simulink model "ConfiguredVirtualVehicleModel"  (R2025b)
settings: Solver=ode14x  StartTime=0  StopTime=inf  FixedStep=.001  RelTol=1e-2  EnableMultiTasking=on
StopFcn:
  | %toc
undefined symbols (not defined in the file or in its folder): CtrlTcuInitGear, DriverPreviewDist, EnvAbsPrs, EnvAirTemp, EnvGrvty, EnvNomFrictionScaling, EnvNominalGrade, EnvWindVelX, EnvWindVelY, EnvWindVelZ, MotoFrmInert, MotoFrmLngth, MotoFrmMass, MotoLowrFrntFrkMass, MotoRearArmLngth, MotoRearArmMass, MotoUpprFrntFrkMass, PlntEngTqMax, RiderMass, Sim3dSensor, trackData
libraries: sm_lib x12, simulink x11, nesl_utility x8, sim3dgroundtruthsensorlib x2, autolibshared x2, vehdynlibdriver x2, instrumentseriallib x2, sharedtransform x1, vehdynlibviscommon x1, autolibutils x1, vehdynlibscenariocommon x1, vehdynlibsteering x1
(part 2 of 5)

== system ConfiguredVirtualVehicleModel/Server Communication/Performance Calculations ==
  VehSpd : Inport
  FuelVolFlow : Inport  Port=2
  Integrator : Integrator
  Integrator1 : Integrator
  L/100 Km Calc : Product  Inputs=/*
  Product : Product
  Rate Transition3 : RateTransition  Deterministic=off
  Saturation : Saturate  UpperLimit=Inf  LowerLimit=0.001  ZeroCross=off
  Saturation1 : Saturate  UpperLimit=Inf  LowerLimit=1e-3  ZeroCross=off
  Signal Specification5 : SignalSpecification  Unit=m/s
  Sqrt : Sqrt
  US MPG Calc : Product  Inputs=*/
  Unit Conversion5 : UnitConversion
  m to 100Km : Gain  Gain=1/1000/100
  m to mile : Gain  Gain=0.000621371
  m^3 to L : Gain  Gain=1000
  m^3 to US Gal : Gain  Gain=264.172
  US MPG : Outport  VectorParamsAs1DForOutWhenUnconnected=off
  L/100Km : Outport  Port=2  VectorParamsAs1DForOutWhenUnconnected=off
  wires:
  m^3 to US Gal/1 -> Saturation1/1
  m^3 to L/1 -> L/100 Km Calc/2
  Integrator/1 -> m to mile/1, m to 100Km/1
  m to mile/1 -> US MPG Calc/1
  Integrator1/1 -> m^3 to US Gal/1, m^3 to L/1
  Saturation/1 -> L/100 Km Calc/1
  m to 100Km/1 -> Saturation/1
  L/100 Km Calc/1 -> L/100Km/1  "L/100Km"
  US MPG Calc/1 -> Rate Transition3/1
  Saturation1/1 -> US MPG Calc/2
  Rate Transition3/1 -> US MPG/1  "US MPG"
  FuelVolFlow/1 -> Integrator1/1
  Sqrt/1 -> Integrator/1
  Product/1 -> Sqrt/1
  Signal Specification5/1 -> Product/2, Product/1
  Unit Conversion5/1 -> Signal Specification5/1
  VehSpd/1 -> Unit Conversion5/1

== system ConfiguredVirtualVehicleModel/Visualization/DataLogging ==
  VehFdbk : Inport
  Bus Selector : BusSelector  OutputSignals=Body.Genrl.Vel.xdot,Body.Genrl.Ang.thetafrm,Body.Genrl.AngVel.thetafrmdot,RearArm.Genrl.Ang.thetara,Body.BdyFrm.Cg.Acc.ax,Body.BdyFrm.Cg.Acc.ay,RearArm.Genrl.AngVel.thetaradot,Driveline.EngSpd,Wheels.RearTire.Omega
  Terminator{,1..8} (9 alike) : Terminator
  wires:
  Bus Selector/7 -> Terminator6/1  "<thetaradot>"
  VehFdbk/1 -> Bus Selector/1
  Bus Selector/6 -> Terminator5/1  "<ay>"
  Bus Selector/5 -> Terminator4/1  "<ax>"
  Bus Selector/1 -> Terminator/1  "<xdot>"
  Bus Selector/4 -> Terminator3/1  "<thetara>"
  Bus Selector/3 -> Terminator2/1  "<thetafrmdot>"
  Bus Selector/2 -> Terminator1/1  "<thetafrm>"
  Bus Selector/8 -> Terminator7/1  "<EngSpd>"
  Bus Selector/9 -> Terminator8/1  "<Omega>"

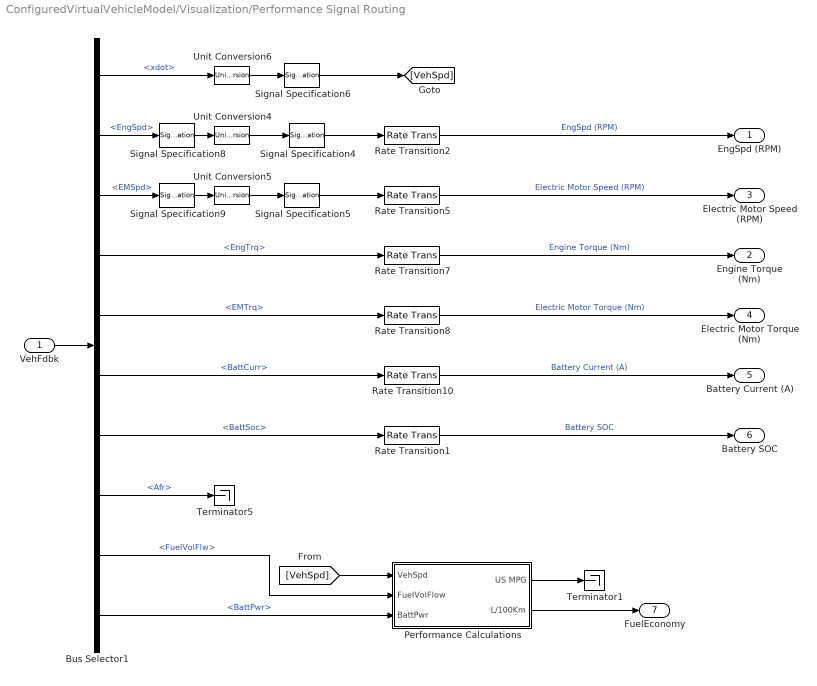
== system ConfiguredVirtualVehicleModel/Visualization/Performance Signal Routing ==
  VehFdbk : Inport
  Bus Selector1 : BusSelector  OutputSignals=Body.BdyFrm.Cg.Vel.xdot,Driveline.EngSpd,Driveline.EMSpd,Engine.EngTrq,ElecMachine.EMTrq,Battery.BattCurr,Battery.BattSoc,Engine.EngineInfo.Afr,Engine.EngineInfo.FuelVolFlw,Battery.BattPwr
  Performance Calculations : Subsystem
  Rate Transition{1..2,5,7..8,10} (6 alike) : RateTransition  Deterministic=off
  Signal Specification4 : SignalSpecification  Unit=rpm
  Signal Specification5 : SignalSpecification  Unit=rpm
  Signal Specification6 : SignalSpecification  Unit=mph
  Signal Specification8 : SignalSpecification  Unit=rad/s
  Signal Specification9 : SignalSpecification  Unit=rad/s
  Terminator1 : Terminator
  Terminator5 : Terminator
  Unit Conversion4 : UnitConversion
  Unit Conversion5 : UnitConversion
  Unit Conversion6 : UnitConversion
  EngSpd (RPM) : Outport
  Engine Torque (Nm) : Outport  Port=2
  Electric Motor Speed (RPM) : Outport  Port=3
  Electric Motor Torque (Nm) : Outport  Port=4
  Battery Current (A) : Outport  Port=5
  Battery SOC : Outport  Port=6
  FuelEconomy : Outport  Port=7
  wires:
  Signal Specification4/1 -> Rate Transition2/1
  Performance Calculations/2(L/100Km) -> FuelEconomy/1
  Bus Selector1/4 -> Rate Transition7/1  "<EngTrq>"
  Bus Selector1/7 -> Rate Transition1/1  "<BattSoc>"
  Signal Specification6/1 -> [VehSpd]
  Bus Selector1/9 -> Performance Calculations/2(FuelVolFlow)  "<FuelVolFlw>"
  Bus Selector1/5 -> Rate Transition8/1  "<EMTrq>"
  Bus Selector1/10 -> Performance Calculations/3(BattPwr)  "<BattPwr>"
  Bus Selector1/2 -> Signal Specification8/1  "<EngSpd>"
  Rate Transition7/1 -> Engine Torque (Nm)/1  "Engine Torque (Nm)"
  Unit Conversion6/1 -> Signal Specification6/1
  Bus Selector1/6 -> Rate Transition10/1  "<BattCurr>"
  Signal Specification5/1 -> Rate Transition5/1
  Unit Conversion5/1 -> Signal Specification5/1
  Unit Conversion4/1 -> Signal Specification4/1
  Signal Specification9/1 -> Unit Conversion5/1
  Signal Specification8/1 -> Unit Conversion4/1
  Bus Selector1/8 -> Terminator5/1  "<Afr>"
  Rate Transition2/1 -> EngSpd (RPM)/1  "EngSpd (RPM)"
  Bus Selector1/3 -> Signal Specification9/1  "<EMSpd>"
  [VehSpd] -> Performance Calculations/1(VehSpd)
  Bus Selector1/1 -> Unit Conversion6/1  "<xdot>"
  Rate Transition8/1 -> Electric Motor Torque (Nm)/1  "Electric Motor Torque (Nm)"
  Rate Transition5/1 -> Electric Motor Speed (RPM)/1  "Electric Motor Speed (RPM)"
  VehFdbk/1 -> Bus Selector1/1
  Rate Transition1/1 -> Battery SOC/1  "Battery SOC"
  Rate Transition10/1 -> Battery Current (A)/1  "Battery Current (A)"
  Performance Calculations/1(US MPG) -> Terminator1/1

== system ConfiguredVirtualVehicleModel/Environment/Friction/Constant Friction ==
  Friction Scaling : Constant  Value=ones(2,1).*EnvNomFrictionScaling  SampleTime=0
  FricCoeffLambda : Outport
  wires:
  Friction Scaling/1 -> FricCoeffLambda/1

== system ConfiguredVirtualVehicleModel/Environment/Friction/Varying Friction ==
  MotoFdbk : Inport
  Bus Selector1 : BusSelector  OutputSignals=Whl.Genrl.Frnt.Cp.Disp.x,Whl.Genrl.Rear.Cp.Disp.x,Whl.Genrl.Frnt.Cp.Disp.y,Whl.Genrl.Rear.Cp.Disp.y
  Bus Selector2 : BusSelector  OutputSignals=Body.InertFrm.Cg.Disp
  Road Track Friction : Subsystem  mask(Road Track Friction){surface_popup=Split friction coefficient scaling factor, lambda_g=EnvNomFrictionScaling, lambda_r=.6, r_x0=175, r_y0=-100, r_xw=1000, r_yw=500, aMode=2}
      mask prompts: surface_popup "vdynblks:vehdynManFriction:blkPrm_surface_popup"; lambda_g "vdynblks:vehdynManFriction:blkPrm_lambda_g"; lambda_r "vdynblks:vehdynManFriction:blkPrm_lambda_r"; r_x0 "vdynblks:vehdynManFriction:blkPrm_r_x0"; r_y0 "vdynblks:vehdynManFriction:blkPrm_r_y0"; r_xw "vdynblks:vehdynManFriction:blkPrm_r_xw"; r_yw "vdynblks:vehdynManFriction:blkPrm_r_yw"
      mask init:
      | % Scaling factor for the friction coefficient around the rectangular region
      | mutable = [lambda_g, lambda_g, lambda_g, lambda_g;
      |            lambda_g, lambda_r, lambda_r, lambda_g; 
      |            lambda_g, lambda_r, lambda_r, lambda_g; 
      |            lambda_g, lambda_g, lambda_g, lambda_g ];
      |        
      | 
      | % The step is distance between breakpoint near the boundary of high and
      | % low friction coefficient
      | 
      | step = 0.01 ; 
      | 
      | % In the mask initialization, xbr and ybr breakpoints are with respect to
      | % Body fixed coordinate system. At time t=0, xbr and ybr breakpoints
      | % updates to Earth (Inertial) Fixed coordinate system. The breakpoints for
      | % the lookup table are added via inputs.
      | 
      | xbr = [(r_x0 - step) , (r_x0 + step), (r_x0 + r_xw - step) , (r_x0 + r_xw + step) ];
      | ybr = [(r_y0 - step) , (r_y0 + step), (r_y0 + r_yw - step) , (r_y0 + r_yw + step) ];
      | 
      | 
      | % To check if the created track is split mu or constant mu
      | 
      | surface_popup = get_param(gcb, 'surface_popup');
      | 
      | if strcmp(surface_popup, 'Split friction coefficient scaling factor')
      |     SplitLambdaTrck = 1;
      | elseif strcmp(surface_popup, 'Constant friction coefficient scaling factor')
      |     SplitLambdaTrck = 0;
      | end
      mask Help: eval('vdynblkshelp(''vdynblkstrack'')');
      mask TypeOptions surface_popup: vdynblks:vehdynManFriction:blkCmb_surface_popup_c1 | vdynblks:vehdynManFriction:blkCmb_surface_popup_c2
      mask Callback surface_popup:
      | surface_popup = get_param(gcb, 'surface_popup');
      | m = Simulink.Mask.get(gcb);
      | 
      | lambda_g = m.getParameter('lambda_g');
      | lambda_r = m.getParameter('lambda_r');
      | r_x0 = m.getParameter('r_x0');
      | r_y0 = m.getParameter('r_y0');
      | r_xw = m.getParameter('r_xw');
      | r_yw = m.getParameter('r_yw');
      | %track_view = m.getParameter('track_view');
      | 
      | 
      | if strcmp(surface_popup, 'Split friction coefficient scaling factor')
      |     lambda_g.Visible = 'on';
      |     lambda_r.Visible = 'on';
      |     r_x0.Visible = 'on';
      |     r_y0.Visible = 'on';
      |     r_xw.Visible = 'on';
      |     r_yw.Visible = 'on';
      |     %track_view.Visible = 'on';
      | 
      | elseif strcmp(surface_popup,'Constant friction coefficient scaling factor')
      |     lambda_g.Visible = 'on';
      |     lambda_r.Visible = 'off';
      |     r_x0.Visible = 'off';
      |     r_y0.Visible = 'off';
      |     r_xw.Visible = 'off';
      |     r_yw.Visible = 'off';
      |     %track_view.Visible = 'off';
      | end
      | [~]=autosharedicon('autolibutils',gcb,0);
      mask DialogControl DescGroupVar Prompt: Road Track Friction
      mask DialogControl DescTextVar Prompt: vdynblks:vehdynManFriction:blkDesc
      mask DialogControl surface_popup Prompt: Type of surface:
      mask DialogControl lambda_g Prompt: Scaling factor for the friction coefficient of ground, lambda_g :
      mask DialogControl lambda_r Prompt: Scaling factor for the friction coefficient of rectangular surface, lambda_r :
      mask DialogControl r_x0 Prompt: X coordinate of lower left corner of rectangular surface, r_x0 [m]:
      mask DialogControl r_y0 Prompt: Y coordinate of lower left corner of rectangular surface, r_y0 [m]:
      mask DialogControl r_xw Prompt: Rectangular surface width in X direction, r_xw [m]:
      mask DialogControl r_yw Prompt: Rectangular surface width in Y direction, r_yw [m]:
  Wheel Coordinates : Subsystem
  FricCoeffLambda : Outport
  wires:
  Wheel Coordinates/1(XWhl) -> Road Track Friction/1(XWhl)
  MotoFdbk/1 -> Bus Selector2/1, Bus Selector1/1
  Wheel Coordinates/2(YWhl) -> Road Track Friction/2(YWhl)
  Road Track Friction/1(FricCoeffLambda) -> FricCoeffLambda/1
  Bus Selector2/1 -> Road Track Friction/3(Cg)  "<Disp>"
  Bus Selector1/1 -> Wheel Coordinates/1(FrntAxlX)  "<x>"
  Bus Selector1/2 -> Wheel Coordinates/2(RearAxlX)  "<x>"
  Bus Selector1/3 -> Wheel Coordinates/3(FrntAxlY)  "<y>"
  Bus Selector1/4 -> Wheel Coordinates/4(RearAxlY)  "<y>"

== system ConfiguredVirtualVehicleModel/Environment/Ground Feedback/3D Engine ==
  Friction : Inport
  WheelFdbk : Inport  Port=2
  3D Engine Source : Subsystem  Variant=on  VariantControl=Choice  mask(Terrain Source){terrType=Single point}
      mask prompts: terrType "Terrain feedback type:"
      mask help:
      | This variant subsystem provides the option for:
      | - a single point of contact for each wheel with minimal post-processing ideal for smooth surfaces and maximum run-time performance.
      | - multiple points of contact per wheel which may be used when interested in non-smooth terrain at a higher computational cost and requires Vehicle Dynamics Blockset.
      mask TypeOptions terrType: Single point | Multiple points
  Bus Creator2 : BusCreator  Inputs=2
  Bus Creator3 : BusCreator  Inputs=3
  Demux1 : Demux  Outputs=2
  Signal Specification1 : SignalSpecification  Unit=1
  Ground : Outport  VectorParamsAs1DForOutWhenUnconnected=off
  wires:
  3D Engine Source/2(DCM) -> Bus Creator3/2  "DCM"
  3D Engine Source/1(z) -> Bus Creator3/1  "z"
  WheelFdbk/1 -> 3D Engine Source/1(WheelFdbk)
  Friction/1 -> Signal Specification1/1
  Bus Creator3/1 -> Ground/1
  Bus Creator2/1 -> Bus Creator3/3  "mu"
  Demux1/2 -> Bus Creator2/2  "mu_R"
  Demux1/1 -> Bus Creator2/1  "mu_F"
  Signal Specification1/1 -> Demux1/1

== system ConfiguredVirtualVehicleModel/Environment/Ground Feedback/Constant ==
  Friction : Inport
  Bus Creator : BusCreator  Inputs=2
  Bus Creator2 : BusCreator  Inputs=2
  Bus Creator3 : BusCreator  Inputs=3
  Constant1 : Constant  Value=zeros(2,1)
  Constant2 : Constant  Value=repmat(eye(3),1,1,2)  SampleTime=-1
  Demux : Demux  Outputs=2
  Demux1 : Demux  Outputs=2
  Signal Specification : SignalSpecification  Unit=m
  Signal Specification1 : SignalSpecification  Unit=1
  Ground : Outport  VectorParamsAs1DForOutWhenUnconnected=off
  wires:
  Constant1/1 -> Signal Specification/1
  Signal Specification/1 -> Demux/1
  Demux/1 -> Bus Creator/1  "G_F_z"
  Demux/2 -> Bus Creator/2  "G_R_z"
  Bus Creator/1 -> Bus Creator3/1  "z"
  Demux1/1 -> Bus Creator2/1  "mu_F"
  Demux1/2 -> Bus Creator2/2  "mu_R"
  Bus Creator2/1 -> Bus Creator3/3  "mu"
  Friction/1 -> Signal Specification1/1
  Signal Specification1/1 -> Demux1/1
  Bus Creator3/1 -> Ground/1
  Constant2/1 -> Bus Creator3/2  "DCM"

== system ConfiguredVirtualVehicleModel/Motorcycle Vehicle/Body, Steer, Suspension, Wheels/Body, Steer, Suspension, Wheels ==
  WindXYZ : Inport
  BrkPrs : Inport  Port=2
  MDrvSprtR : Inport  Port=3
  MDrvArmR : Inport  Port=4
  MDrvFrm : Inport  Port=5
  ScaleFactrs : Inport  Port=6
  SteerCmd : Inport  Port=7
  In_Plane_ModelArchitecture : Subsystem  VariantControl=In_Plane_ModelArchitecture  ReferencedSubsystem=In_Plane_ModelArchitecture
  Moto : Outport
  Wheels : Outport  Port=2

== system ConfiguredVirtualVehicleModel/Motorcycle Vehicle/Body, Steer, Suspension, Wheels/Chassis Input ==
  Env : Inport
  Driveline : Inport  Port=2
  Rider : Inport  Port=3
  Bus Selector : BusSelector  OutputSignals=SteerFdbk
  Bus Selector2 : BusSelector  OutputSignals=Wind,Gnd.mu
  Bus Selector4 : BusSelector  OutputSignals=BrkPrs,Info.ChainInfo.MDrvSprtR,Info.MDrvArmR,Info.MDrvFrm
  Bus to Vector : BusToVector
  Wind : Outport  VectorParamsAs1DForOutWhenUnconnected=off
  BrkPrs : Outport  Port=2  VectorParamsAs1DForOutWhenUnconnected=off
  MDrvSprtR : Outport  Port=3  VectorParamsAs1DForOutWhenUnconnected=off
  MDrvArmR : Outport  Port=4  VectorParamsAs1DForOutWhenUnconnected=off
  MDrvFrm : Outport  Port=5  VectorParamsAs1DForOutWhenUnconnected=off
  ScaleFactrs : Outport  Port=6  VectorParamsAs1DForOutWhenUnconnected=off
  SteerCmd : Outport  Port=7  VectorParamsAs1DForOutWhenUnconnected=off
  wires:
  Env/1 -> Bus Selector2/1
  Bus Selector2/1 -> Wind/1  "<Wind>"
  Driveline/1 -> Bus Selector4/1
  Bus Selector4/4 -> MDrvFrm/1  "<MDrvFrm>"
  Bus Selector4/3 -> MDrvArmR/1  "<MDrvArmR>"
  Bus Selector4/2 -> MDrvSprtR/1  "<MDrvSprtR>"
  Bus Selector4/1 -> BrkPrs/1  "<BrkPrs>"
  Bus Selector2/2 -> Bus to Vector/1  "<mu>"
  Bus to Vector/1 -> ScaleFactrs/1
  Rider/1 -> Bus Selector/1
  Bus Selector/1 -> SteerCmd/1  "<SteerFdbk>"

== system ConfiguredVirtualVehicleModel/Motorcycle Vehicle/Body, Steer, Suspension, Wheels/Chassis Output ==
  Moto : Inport
  Wheels : Inport  Port=2
  Out Bus Element4 : Outport  PortName=MotoFdbk
  Out Bus Element1 : Outport  Port=2  PortName=WheelsFdbk
  wires:
  Moto/1 -> Out Bus Element4/1
  Wheels/1 -> Out Bus Element1/1

== system ConfiguredVirtualVehicleModel/Motorcycle Vehicle/Control Feedback/Variant Subsystem ==
  note: 1) Add Subsystem or Model blocks as valid variant choices.
      | 2) You cannot connect blocks at this level. At simulation, connectivity is automatically
      | determined, based on the active variant and port name matching.
  MotoFdbk : Inport
  IMU_Sensor : Subsystem  VariantControl=IMU_Sensor  ReferencedSubsystem=IMU_Sensor
  No_IMU_Sensor : Subsystem  VariantControl=No_IMU_Sensor  ReferencedSubsystem=No_IMU_Sensor
  IMU : Outport

== system ConfiguredVirtualVehicleModel/Motorcycle Vehicle/Hand Levers and Pedals/Hand Levers and Pedals ==
  note: Placeholder for introducing faults, detailed actuator behavior,
      | interactions of other systems with a human interface such
      | as changes in power steering and braking assistance.
  SteerCmd : Inport
  AccCmd : Inport  Port=2
  DecelCmd : Inport  Port=3
  GearCmd : Inport  Port=4
  BrkPrs : Inport  Port=5
  StrWhlTrq : Inport  Port=6
  Brake Pedal : Subsystem
  Dead Zone3 : DeadZone  LowerValue=-.01  UpperValue=.01  ZeroCross=off
  Terminator : Terminator
  Terminator1 : Terminator
  Twist2Acc : Lookup_n-D  NumberOfTableDimensions=1  BreakpointsForDimension1=[0 1]  Table=[0 1]  ExtrapMethod=Clip  InternalRulePriority=Speed  RndMeth=Simplest
  SteerFdbk : Outport
  AccFdbk : Outport  Port=2
  DecelFdbk : Outport  Port=3
  GearFdbk : Outport  Port=4
  wires:
  SteerCmd/1 -> Dead Zone3/1
  DecelCmd/1 -> Brake Pedal/1(DecelCmd)
  GearCmd/1 -> GearFdbk/1
  BrkPrs/1 -> Terminator/1
  StrWhlTrq/1 -> Terminator1/1
  Brake Pedal/1(DecelFdbk) -> DecelFdbk/1
  Dead Zone3/1 -> SteerFdbk/1
  AccCmd/1 -> Twist2Acc/1
  Twist2Acc/1 -> AccFdbk/1

== system ConfiguredVirtualVehicleModel/Motorcycle Vehicle/Hand Levers and Pedals/Pedal Cluster Input ==
  Rider : Inport
  Driveline : Inport  Port=2
  Bus Selector : BusSelector  OutputSignals=SteerCmd,AccelCmd,DecelCmd,GearCmd
  Bus Selector1 : BusSelector  OutputSignals=EMSpd
  Constant : Constant  Value=0
  SteerCmd : Outport  VectorParamsAs1DForOutWhenUnconnected=off
  AccelCmd : Outport  Port=2  VectorParamsAs1DForOutWhenUnconnected=off
  DecelCmd : Outport  Port=3  VectorParamsAs1DForOutWhenUnconnected=off
  GearCmd : Outport  Port=4  VectorParamsAs1DForOutWhenUnconnected=off
  BrkPrs : Outport  Port=5  VectorParamsAs1DForOutWhenUnconnected=off
  StrWhlTrq : Outport  Port=6  VectorParamsAs1DForOutWhenUnconnected=off
  wires:
  Bus Selector/2 -> AccelCmd/1  "<AccelCmd>"
  Rider/1 -> Bus Selector/1
  Bus Selector/3 -> DecelCmd/1  "<DecelCmd>"
  Bus Selector/4 -> GearCmd/1  "<GearCmd>"
  Bus Selector/1 -> SteerCmd/1  "<SteerCmd>"
  Driveline/1 -> Bus Selector1/1
  Bus Selector1/1 -> BrkPrs/1  "<EMSpd>"
  Constant/1 -> StrWhlTrq/1

== system ConfiguredVirtualVehicleModel/Motorcycle Vehicle/Hand Levers and Pedals/Pedal Cluster Output ==
  SteerFdbk : Inport
  AccFdbk : Inport  Port=2
  DecelFdbk : Inport  Port=3
  GearFdbk : Inport  Port=4
  Bus Creator1 : BusCreator  Inputs=4
  Signal Specification : SignalSpecification  Unit=N*m
  Signal Specification1 : SignalSpecification  Unit=1
  Signal Specification2 : SignalSpecification  Unit=1
  Signal Specification3 : SignalSpecification  Unit=1
  OperatorFdbk : Outport
  wires:
  Signal Specification1/1 -> Bus Creator1/2  "AccFdbk"
  Signal Specification3/1 -> Bus Creator1/4  "GearFdbk"
  AccFdbk/1 -> Signal Specification1/1
  DecelFdbk/1 -> Signal Specification2/1
  GearFdbk/1 -> Signal Specification3/1
  Signal Specification/1 -> Bus Creator1/1  "SteerFdbk"
  SteerFdbk/1 -> Signal Specification/1
  Bus Creator1/1 -> OperatorFdbk/1
  Signal Specification2/1 -> Bus Creator1/3  "DecelFdbk"

== system ConfiguredVirtualVehicleModel/Motorcycle Vehicle/Propulsion System/Actuators ==
  note: 1) Add Subsystem or Model blocks as valid variant choices.
      | 2) You cannot connect blocks at this level. At simulation, connectivity is automatically
      | determined, based on the active variant and port name matching.
  TrqCmd : Inport
  EngSpd : Inport  Port=2
  EMTrqCmd : Inport  Port=3
  EMSpd : Inport  Port=4
  AmbTemp : Inport  Port=5
  MotoMappedEngine : Subsystem  VariantControl=MotoMappedEngine  ReferencedSubsystem=MotoMappedEngine
  Eng : Outport
  Battery : Outport  Port=2
  ElecMachine : Outport  Port=3

== system ConfiguredVirtualVehicleModel/Motorcycle Vehicle/Propulsion System/Electrical System Input ==
  Cntrl : Inport
  Driveline : Inport  Port=2
  Env : Inport  Port=3
  Bus Selector : BusSelector  OutputSignals=VCU.EMTrqCmd
  Bus Selector1 : BusSelector  OutputSignals=EMSpd
  Bus Selector2 : BusSelector  OutputSignals=Temp
  First Order Hold : FirstOrderHold  ErrorTolerance=inf
  EMTrqCmd : Outport  VectorParamsAs1DForOutWhenUnconnected=off
  EMSpd : Outport  Port=2  VectorParamsAs1DForOutWhenUnconnected=off
  AmbTemp : Outport  Port=3  VectorParamsAs1DForOutWhenUnconnected=off
  wires:
  Cntrl/1 -> Bus Selector/1
  Bus Selector/1 -> First Order Hold/1  "<EMTrqCmd>"
  Bus Selector1/1 -> EMSpd/1  "<EMSpd>"
  Env/1 -> Bus Selector2/1
  Bus Selector2/1 -> AmbTemp/1  "<Temp>"
  Driveline/1 -> Bus Selector1/1
  First Order Hold/1 -> EMTrqCmd/1

== system ConfiguredVirtualVehicleModel/Motorcycle Vehicle/Propulsion System/Engine Input ==
  Cntrl : Inport
  Driveline : Inport  Port=2
  Bus Selector : BusSelector  OutputSignals=ECU.EngTrqCmd
  Bus Selector1 : BusSelector  OutputSignals=EngSpd
  First Order Hold : FirstOrderHold  OutputAlgorithm=Fast (Minimize Error)  ErrorTolerance=.001
  Rate Transition : RateTransition  OutPortSampleTime=0.001
  EngTrqCmd : Outport  VectorParamsAs1DForOutWhenUnconnected=off
  EngSpd : Outport  Port=2  VectorParamsAs1DForOutWhenUnconnected=off
  wires:
  Driveline/1 -> Bus Selector1/1
  Cntrl/1 -> Bus Selector/1
  Bus Selector/1 -> Rate Transition/1  "<EngTrqCmd>"
  Bus Selector1/1 -> EngSpd/1  "<EngSpd>"
  First Order Hold/1 -> EngTrqCmd/1
  Rate Transition/1 -> First Order Hold/1

== system ConfiguredVirtualVehicleModel/Motorcycle Vehicle/Transmission, Driveline and Brakes/Brake Hydraulics ==
  BrkPrsCmd : Inport
  Front Bias : Constant
  Gain4 : Gain  Gain=8e6
  Mux : Mux  Inputs=2
  Product : Product
  Rear Bias : Constant  Value=.6
  Valve : autolibutils/Cont LPF  wc=20*2*pi  AbsoluteTolerance=auto  aMode=2
  BrkPrs : Outport  VectorParamsAs1DForOutWhenUnconnected=off
  wires:
  Valve/1 -> Product/2
  Gain4/1 -> BrkPrs/1
  BrkPrsCmd/1 -> Valve/1
  Front Bias/1 -> Mux/1
  Rear Bias/1 -> Mux/2
  Product/1 -> Gain4/1
  Mux/1 -> Product/1

== system ConfiguredVirtualVehicleModel/Motorcycle Vehicle/Transmission, Driveline and Brakes/Driveline Input ==
  Cntrl : Inport
  EngTrqCmd : Inport  Port=2
  Wheels : Inport  Port=3
  Moto : Inport  Port=4
  EMTrqCmd : Inport  Port=5
  Bus Selector : BusSelector  OutputSignals=EngTrq
  Bus Selector1 : BusSelector  OutputSignals=EMTrq
  Bus Selector2 : BusSelector  OutputSignals=RearTire.Fx,RearTire.MBrk,RearTire.Omegadot
  Bus Selector3 : BusSelector  OutputSignals=Transmission.GearCmd,VCU.VcuBrkPrsCmd
  Bus Selector5 : BusSelector  OutputSignals=Frame.Genrl.Ang.thetafrm,RearArm.Genrl.Ang.thetara
  Data Type Conversion : DataTypeConversion  SaturateOnIntegerOverflow=off  RndMeth=Floor
  First Order Hold1 : FirstOrderHold  OutputAlgorithm=Fast (Minimize Error)  ErrorTolerance=.001
  First Order Hold2 : FirstOrderHold  InitialOutput=CtrlTcuInitGear  ErrorTolerance=.5
  EngTrq : Outport  VectorParamsAs1DForOutWhenUnconnected=off
  GearCmd : Outport  Port=2  VectorParamsAs1DForOutWhenUnconnected=off
  FCpR. : Outport  Port=3  VectorParamsAs1DForOutWhenUnconnected=off
  ThetaFrm. : Outport  Port=4  VectorParamsAs1DForOutWhenUnconnected=off
  ThetaArmR. : Outport  Port=5  VectorParamsAs1DForOutWhenUnconnected=off
  MBrkR. : Outport  Port=6  VectorParamsAs1DForOutWhenUnconnected=off
  AngAWhlR. : Outport  Port=7  VectorParamsAs1DForOutWhenUnconnected=off
  EMTrq : Outport  Port=8  VectorParamsAs1DForOutWhenUnconnected=off
  BrkPrsCmd : Outport  Port=9  VectorParamsAs1DForOutWhenUnconnected=off
  wires:
  Wheels/1 -> Bus Selector2/1
  Moto/1 -> Bus Selector5/1
  Bus Selector2/3 -> AngAWhlR./1  "<Omegadot>"
  Bus Selector2/2 -> MBrkR./1  "<MBrk>"
  Bus Selector2/1 -> FCpR./1  "<Fx>"
  Bus Selector5/2 -> ThetaArmR./1  "<thetara>"
  Bus Selector5/1 -> ThetaFrm./1  "<thetafrm>"
  EngTrqCmd/1 -> Bus Selector/1
  EMTrqCmd/1 -> Bus Selector1/1
  Bus Selector3/2 -> First Order Hold1/1  "<VcuBrkPrsCmd>"
  Bus Selector3/1 -> Data Type Conversion/1  "<GearCmd>"
  Cntrl/1 -> Bus Selector3/1
  Bus Selector/1 -> EngTrq/1  "<EngTrq>"
  Bus Selector1/1 -> EMTrq/1  "<EMTrq>"
  First Order Hold1/1 -> BrkPrsCmd/1
  Data Type Conversion/1 -> First Order Hold2/1
  First Order Hold2/1 -> GearCmd/1

== system ConfiguredVirtualVehicleModel/Motorcycle Vehicle/Transmission, Driveline and Brakes/Driveline Output ==
  EngSpd : Inport
  Gear : Inport  Port=2
  Info : Inport  Port=3
  EMSpd : Inport  Port=4
  BrkPrs : Inport  Port=5
  Bus Creator1 : BusCreator  Inputs=7
  Ground{,1..3} (4 alike) : Ground
  Mux : Mux  Inputs=2
  Mux1 : Mux  Inputs=2
  Signal Specification7 : SignalSpecification  Unit=Pa  Dimensions=2
  Driveline : Outport  VectorParamsAs1DForOutWhenUnconnected=off
  wires:
  Bus Creator1/1 -> Driveline/1  "Driveline"
  EngSpd/1 -> Bus Creator1/3  "EngSpd"
  EMSpd/1 -> Bus Creator1/2  "EMSpd"
  Gear/1 -> Bus Creator1/4  "Gear"
  Info/1 -> Bus Creator1/7  "Info"
  Mux/1 -> Bus Creator1/6  "AxlTrq"
  Mux1/1 -> Bus Creator1/5  "PropShftSpd"
  Ground3/1 -> Mux/2
  Ground2/1 -> Mux/1
  Ground/1 -> Mux1/1
  Ground1/1 -> Mux1/2
  BrkPrs/1 -> Signal Specification7/1
  Signal Specification7/1 -> Bus Creator1/1  "BrkPrs"

== system ConfiguredVirtualVehicleModel/Motorcycle Vehicle/Transmission, Driveline and Brakes/Transmission and Driveline ==
  EngTrq : Inport
  GearCmd : Inport  Port=2
  FCpR : Inport  Port=3
  ThetaFrm : Inport  Port=4
  ThetaArmR : Inport  Port=5
  MBrkR : Inport  Port=6
  AngAWhlR : Inport  Port=7
  EMTrq : Inport  Port=8
  Driveline : Subsystem  Variant=on  VariantChoicesSpecifier={'Chain_Drive'}  VariantControlMode=label  VariantControl=Choice  LabelModeActiveChoice=Chain_Drive
  Transmission : Subsystem  Variant=on  VariantChoicesSpecifier={'ConventionalMotorcycle'}  VariantControlMode=label  VariantControl=Choice  LabelModeActiveChoice=ConventionalMotorcycle
  EngSpd : Outport
  Gear : Outport  Port=2
  Info : Outport  Port=3
  EMSpd : Outport  Port=4
  wires:
  EngTrq/1 -> Transmission/1(EngTrq)
  GearCmd/1 -> Transmission/2(GearCmd)
  FCpR/1 -> Driveline/1(FCpR)
  ThetaFrm/1 -> Driveline/2(ThetaFrm)
  ThetaArmR/1 -> Driveline/3(ThetaArmR)
  MBrkR/1 -> Driveline/4(MBrkR)
  AngAWhlR/1 -> Driveline/5(AngAWhlR)
  EMTrq/1 -> Transmission/3(EMTrq)
  Driveline/2(DrvSprktSpd) -> Transmission/4(DrvSprktSpd)
  Transmission/4(DrvSprktTrq) -> Driveline/6(DrvSprktTrq)
  Driveline/1(Info) -> Info/1
  Transmission/1(EngSpd) -> EngSpd/1
  Transmission/2(Gear) -> Gear/1
  Transmission/3(EMSpd) -> EMSpd/1

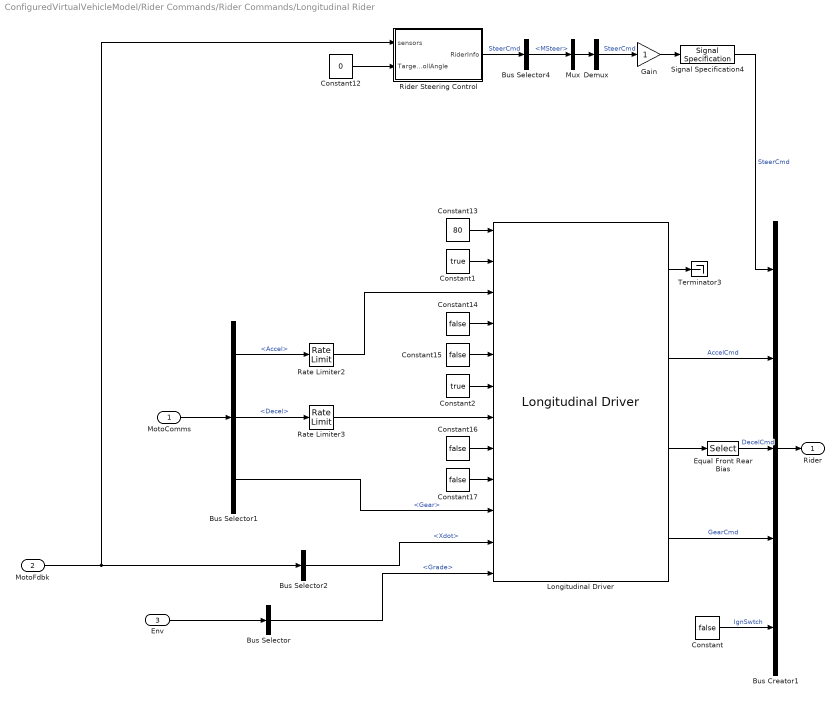
== system ConfiguredVirtualVehicleModel/Rider Commands/Rider Commands/Longitudinal Rider ==
  MotoComms : Inport
  MotoFdbk : Inport  Port=2
  Env : Inport  Port=3
  Bus Creator1 : BusCreator  Inputs=5
  Bus Selector : BusSelector  OutputSignals=Grade
  Bus Selector1 : BusSelector  OutputSignals=Accel,Decel,Gear
  Bus Selector2 : BusSelector  OutputSignals=Body.InertFrm.Cg.Vel.Xdot
  Bus Selector4 : BusSelector  OutputSignals=MSteer
  Constant{,14..17} (5 alike) : Constant  Value=false
  Constant1 : Constant  Value=true
  Constant12 : Constant  Value=0
  Constant13 : Constant  Value=80
  Constant2 : Constant  Value=true
  Demux : Demux  Outputs=1
  Equal Front Rear Bias : Selector  InputPortWidth=1  IndexOptions=Index vector (dialog)  Indices=[1 1]  OutputSizes=1
  Gain : Gain
  Longitudinal Driver : autolibshared/Longitudinal Driver  extAccelOvr=on  extDecelOvr=on  extAccelHld=on  extDecelHld=on  extAccelZero=on  extDecelZero=on  cntrlType=PI  shftType=External  velUnits=m/s  gearOut=on  Kp=5  Ki=5  Kff=.1  Kg=0  VehVelVec=[0 100]  KffVec=[.1 .1]  KpVec=[10 10]  KiVec=[5 5]  KgVec=[0 0]  m=MotoFrmMass+MotoUpprFrntFrkMass+MotoLowrFrntFrkMass+MotoRearArmMass+RiderMass  Kpt=DriverTractiveForce  tau=DriverTimeConst  L=DriverPreviewDist  aR=DriverRollRes  bR=DriverDrivelineRes  cR=DriverAeroRes  g=EnvGrvty  vnom=5  Kaw=1  tauerr=.1  tauPt=2  GearInit=DriverInitialGear  tShift=DriverShiftTime  pdlVec=[0.1 0.4 0.5 0.9]  upShftTbl=|  dwnShftTbl=|  tClutch=.5  tRev=.5  tPark=120  aMode=6  UpGearVec="[0  1  2  3  4  5  6  7  8]"  DownGearVec="[1  2  3  4  5  6  7  8  9]"
      upShftTbl=|
      | [-1 25 42.7198903036173	47.4101666153559	56.5501922484876	82.5161741607935	103.519768418748	161.279652628121	247.919478942182;
      | -1 35 47.2198903036173	51.9101666153559	61.0501922484876	87.0161741607935	108.019768418748	165.779652628121	252.419478942182;
      | -1 40 48.7198903036173	53.4101666153559	62.5501922484876	88.5161741607935	109.519768418748	167.279652628121	253.919478942182;
      | -1 45 54.7198903036173	59.4101666153559	68.5501922484876	94.5161741607935	115.519768418748	173.279652628121	259.919478942182].*0.277778
      dwnShftTbl=|
      | [6 20 38.7198903036173	43.4101666153559	52.5501922484876	78.5161741607935	99.5197684187476	157.279652628121	243.919478942182;
      | 6 30 43.2198903036173	47.9101666153559	57.0501922484876	83.0161741607935	104.019768418748	161.779652628121	248.419478942182;
      | 6 35 44.7198903036173	49.4101666153559	58.5501922484876	84.5161741607935	105.519768418748	163.279652628121	249.919478942182;
      | 6 45 50.7198903036173	55.4101666153559	64.5501922484876	90.5161741607935	111.519768418748	169.279652628121	255.919478942182].*0.277778
  Mux : Mux  Inputs=1
  Rate Limiter2 : RateLimiter  RisingSlewLimit=2  FallingSlewLimit=-5  SampleTimeMode=inherited
  Rate Limiter3 : RateLimiter  RisingSlewLimit=2  FallingSlewLimit=-5  SampleTimeMode=inherited
  Rider Steering Control : Subsystem  mask{RiderControlTypePanel=Roll angle control, TrajectoryTypePanel=Oval, RidTrajContG=0.11, RidTrajContGphi=-21.5, RidTrajContGphid=9, RidTrajContGl=1.7, RidTrajContTD=0.1, RidTrajContTL=0.1, RidRollContGphi=-21.5, RidRollContGphid=9, Trajr=15, Trajl=80, Trajpointdist=1, TrajDatFile='Traj.mat'}
      mask prompts: RiderControlTypePanel "Rider control type:"; TrajectoryTypePanel "Trajectory type:"; RidTrajContG "Gain to determine the Target roll angle, RidContG [rad/m]:"; RidTrajContGphi "Gain to follow the Target trajectory, RidContGphi [Nm/rad]:"; RidTrajContGphid "Gain to prevent the vehicle from tipping over, RidContGphid [Nms/rad]:"; RidTrajContGl "Gain that determines the distance to the look ahead point, RidContGl [s]:"; RidTrajContTD "Time constant for 1st order delay, RidContTD [s]:"; RidTrajContTL "Dead time of rider operation, RidContTL [s]:"; RidRollContGphi "Gain to follow the Target trajectory, RidContGphi [Nm/rad]:"; RidRollContGphid "Gain to prevent the vehicle from tipping over, RidContGphid [Nms/rad]:"; Trajr "Trajectory parameter,Trajr [m]:"; Trajl "Trajectory parameter,Trajl [m]:"; Trajpointdist "Trajpdist [m]:"; TrajDatFile "Trajectory data file:"
      mask init:
      | maskObj = Simulink.Mask.get(gcb);
      | 
      | Type_tmp = maskObj.getParameter('RiderControlTypePanel');
      | Type     = Type_tmp.Value;
      | 
      | TrajGroup = maskObj.getDialogControl('RiderTrajectoryControlParamPanel');
      | RollGroup = maskObj.getDialogControl('RiderRollControlParamPanel');
      | 
      | TrajectoryTypePanel = maskObj.getDialogControl('TrajectoryTypeCont');
      | TargetTrajectoryParamGroup = maskObj.getDialogControl('TargetTrajectoryParamGroup');
      | 
      | GroupAll = maskObj.getDialogControl('RiderControlParamGroup');
      | 
      | switch Type
      |     case 'Roll angle control'
      |     TrajGroup.Visible = 'off';
      |     RollGroup.Visible = 'on';
      |     GroupAll.Visible = 'on';
      |     TrajectoryTypePanel.Visible = 'off';
      |     TargetTrajectoryParamGroup.Visible = 'off';
      |     InputConnector('TargetRollAngle','on');
      |     case 'Target trajectory driving - Look ahead point'
      |     TrajGroup.Visible = 'on';
      |     RollGroup.Visible = 'off';
      |     GroupAll.Visible = 'on';
      |     TrajectoryTypePanel.Visible = 'on';
      |     TargetTrajectoryParamGroup.Visible = 'on';
      |     InputConnector('TargetRollAngle','off','Ground');
      | end
      | 
      | switch Type
      |     case 'Oval'
      | % ------------------------------------------------------------------------%
      | %  Create Trajectory
      | % ------------------------------------------------------------------------%
      | % --- Oval --- %
      | % top part %
      | x_straight1 = -Trajl/2:Trajpointdist:Trajl/2;
      | y_straight1 = x_straight1*0;
      | 
      | % bottom part %
      | x_straight2 = -Trajl/2:Trajpointdist:Trajl/2;
      | y_straight2 = x_straight1*0+2*Trajr;
      | 
      | % right part %
      | theta_corner1 = -pi/2:Trajpointdist/Trajr:pi/2;
      | x_corner1     = Trajr*cos(theta_corner1)+Trajl/2;
      | y_corner1     = Trajr*sin(theta_corner1)+Trajr;
      | 
      | % left part %
      | theta_corner2 = pi/2:Trajpointdist/Trajr:3/2*pi;
      | x_corner2     = Trajr*cos(theta_corner2)-Trajl/2;
      | y_corner2     = Trajr*sin(theta_corner2)+Trajr;
      | 
      | % total %
      | x_oval = [x_straight1, x_corner1(2:end), fliplr(x_straight2), x_corner2(2:end)];
      | y_oval = [y_straight1, y_corner1(2:end), fliplr(y_straight2), y_corner2(2:end)];
      | 
      | trackData(1,:) = x_oval;
      | trackData(2,:) = y_oval;
      | trackData(3,:) = y_oval*0;
      | 
      |     case 'User defined'
      | 
      | TmpTraj = load(TrajDatFile);
      | 
      | trackData(1,:) = TmpTraj.TrajX;
      | trackData(2,:) = -TmpTraj.TrajY;
      | trackData(3,:) = TmpTraj.TrajY*0;
      | 
      | end
      mask Callback RiderControlTypePanel:
      | maskObj = Simulink.Mask.get(gcb);
      | 
      | Type_tmp = maskObj.getParameter('RiderControlTypePanel');
      | Type     = Type_tmp.Value;
      | 
      | TrajGroup = maskObj.getDialogControl('RiderTrajectoryControlParamPanel');
      | RollGroup = maskObj.getDialogControl('RiderRollControlParamPanel');
      | 
      | TrajectoryTypePanel = maskObj.getDialogControl('TrajectoryTypeCont');
      | TargetTrajectoryParamGroup = maskObj.getDialogControl('TargetTrajectoryParamGroup');
      | 
      | GroupAll = maskObj.getDialogControl('RiderControlParamGroup');
      | 
      | switch Type
      |     case 'Roll angle control'
      |     set_param([gcb,'/Rider Steering'],'RiderControlTypePanel','Roll angle control')
      |     TrajGroup.Visible = 'off';
      |     RollGroup.Visible = 'on';
      |     GroupAll.Visible = 'on';
      |     TrajectoryTypePanel.Visible = 'off';
      |     TargetTrajectoryParamGroup.Visible = 'off';
      |     InputConnector('TargetRollAngle','on');
      |     case 'Target trajectory driving - Look ahead point'
      |     set_param([gcb,'/Rider Steering'],'RiderControlTypePanel','Target trajectory driving - Look ahead point')
      |     TrajGroup.Visible = 'on';
      |     RollGroup.Visible = 'off';
      |     GroupAll.Visible = 'on';
      |     TrajectoryTypePanel.Visible = 'on';
      |     TargetTrajectoryParamGroup.Visible = 'on';
      |     InputConnector('TargetRollAngle','off','Ground');
      | end
      mask TypeOptions TrajectoryTypePanel: Oval | User defined
      mask Callback TrajectoryTypePanel:
      | maskObj = Simulink.Mask.get(gcb);
      | 
      | Type_tmp = maskObj.getParameter('TrajectoryTypePanel');
      | Type = Type_tmp.Value;
      | 
      | TargetTrajectoryParamOvalPanel = maskObj.getDialogControl('TargetTrajectoryParamOvalPanel');
      | 
      | TargetTrajectoryParamUserDefinedPanel = maskObj.getDialogControl('TargetTrajectoryParamUserDefinedPanel');
      | 
      | TargetTrajectoryParamGroup = maskObj.getDialogControl('TargetTrajectoryParamGroup');
      | 
      | switch Type
      |     case 'Oval'
      |         set_param([gcb,'/Rider Steering'],'TrajectoryTypePanel','Oval')
      |         % TargetTrajectoryParamGroup.Visible = 'on';
      |         TargetTrajectoryParamOvalPanel.Visible = 'on';
      |         TargetTrajectoryParamUserDefinedPanel.Visible = 'off';
      |     case 'User defined'
      |     set_param([gcb,'/Rider Steering'],'TrajectoryTypePanel','User defined')
      |         % TargetTrajectoryParamGroup.Visible = 'on';
      |         TargetTrajectoryParamOvalPanel.Visible = 'off';
      |         TargetTrajectoryParamUserDefinedPanel.Visible = 'on';
      | end
      mask DialogControl RiderOptionsGroup Prompt: Options
      mask DialogControl RiderTrajectoryControlParamPanel Prompt: Control parameters
      mask DialogControl RiderRollControlParamPanel Prompt: Control parameters
      mask DialogControl TargetTrajectoryParamOvalPanel Prompt: Trajectory parameters
      mask DialogControl OvalTrajConfBtn Prompt: Confirm
      mask DialogControl OvalTrajConfBtn Callback:
      | maskObj = Simulink.Mask.get(gcb);
      | 
      | Trajr_tmp          = maskObj.getParameter('Trajr');
      | Trajr              = str2num(Trajr_tmp.Value);
      | Trajl_tmp          = maskObj.getParameter('Trajl');
      | Trajl              = str2num(Trajl_tmp.Value);
      | Trajpointdist_tmp  = maskObj.getParameter('Trajpointdist');
      | Trajpointdist      = str2num(Trajpointdist_tmp.Value);
      | 
      | % ------------------------------------------------------------------------%
      | %  Create Trajectory
      | % ------------------------------------------------------------------------%
      | % --- Oval --- %
      | % top part %
      | x_straight1 = -Trajl/2:Trajpointdist:Trajl/2;
      | y_straight1 = x_straight1*0;
      | 
      | % bottom part %
      | x_straight2 = -Trajl/2:Trajpointdist:Trajl/2;
      | y_straight2 = x_straight1*0+2*Trajr;
      | 
      | % right part %
      | theta_corner1 = -pi/2:Trajpointdist/Trajr:pi/2;
      | x_corner1     = Trajr*cos(theta_corner1)+Trajl/2;
      | y_corner1     = Trajr*sin(theta_corner1)+Trajr;
      | 
      | % left part %
      | theta_corner2 = pi/2:Trajpointdist/Trajr:3/2*pi;
      | x_corner2     = Trajr*cos(theta_corner2)-Trajl/2;
      | y_corner2     = Trajr*sin(theta_corner2)+Trajr;
      | 
      | % total %
      | x_oval = [x_straight1, x_corner1(2:end), fliplr(x_straight2), x_corner2(2:end)];
      | y_oval = [y_straight1, y_corner1(2:end), fliplr(y_straight2), y_corner2(2:end)];
      | 
      | figure;
      | plot(x_oval, -y_oval);
      | axis equal;
      | grid on;
      | xlabel('Coordinate X [m]');
      | ylabel('Coordinate Y [m]');
      | title('Oval target trajectory');
      | set(gca,'YDir','reverse')
      mask DialogControl TargetTrajectoryParamUserDefinedPanel Prompt: Trajectory parameters
      mask DialogControl UserDefinedTrajConfBtn Prompt: Confirm
      mask DialogControl UserDefinedTrajConfBtn Callback:
      | maskObj = Simulink.Mask.get(gcb);
      | 
      | File_tmp = maskObj.getParameter('TrajDatFile');
      | File     = replace(File_tmp.Value,'''','');
      | 
      | TmpTraj = load(File);
      | 
      | figure;
      | plot(TmpTraj.TrajX, TmpTraj.TrajY);
      | grid on;
      | axis equal;
      | xlabel('Coordinate X [m]');
      | ylabel('Coordinate Y [m]');
      | title('User defined target trajectory');
      | set(gca,'YDir','reverse');
  Signal Specification4 : SignalSpecification  Unit=N*m
  Terminator3 : Terminator
  Rider : Outport  VectorParamsAs1DForOutWhenUnconnected=off
  wires:
  Bus Creator1/1 -> Rider/1
  Longitudinal Driver/3 -> Equal Front Rear Bias/1
  Longitudinal Driver/1 -> Terminator3/1
  MotoComms/1 -> Bus Selector1/1
  Longitudinal Driver/2 -> Bus Creator1/2  "AccelCmd"
  Longitudinal Driver/4 -> Bus Creator1/4  "GearCmd"
  Constant/1 -> Bus Creator1/5  "IgnSwtch"
  Constant2/1 -> Longitudinal Driver/6
  Env/1 -> Bus Selector/1
  Equal Front Rear Bias/1 -> Bus Creator1/3  "DecelCmd"
  Constant1/1 -> Longitudinal Driver/2
  Bus Selector/1 -> Longitudinal Driver/12  "<Grade>"
  Rider Steering Control/1(RiderInfo) -> Bus Selector4/1  "SteerCmd"
  Bus Selector4/1 -> Mux/1  "<MSteer>"
  Signal Specification4/1 -> Bus Creator1/1  "SteerCmd"
  Gain/1 -> Signal Specification4/1
  Demux/1 -> Gain/1  "SteerCmd"
  MotoFdbk/1 -> Rider Steering Control/1(sensors), Bus Selector2/1
  Constant12/1 -> Rider Steering Control/2(TargetRollAngle)
  Mux/1 -> Demux/1
  Constant13/1 -> Longitudinal Driver/1
  Bus Selector2/1 -> Longitudinal Driver/11  "<Xdot>"
  Bus Selector1/3 -> Longitudinal Driver/10  "<Gear>"
  Bus Selector1/1 -> Rate Limiter2/1  "<Accel>"
  Bus Selector1/2 -> Rate Limiter3/1  "<Decel>"
  Constant14/1 -> Longitudinal Driver/4
  Constant15/1 -> Longitudinal Driver/5
  Constant16/1 -> Longitudinal Driver/8
  Constant17/1 -> Longitudinal Driver/9
  Rate Limiter2/1 -> Longitudinal Driver/3
  Rate Limiter3/1 -> Longitudinal Driver/7

== system ConfiguredVirtualVehicleModel/Rider Commands/Rider Commands/Open Loop ==
  MotoFdbk : Inport
  MotoComms : Inport  Port=2
  GearCmd : Inport  Port=3
  Bus Creator1 : BusCreator  Inputs=5
  Bus Selector1 : BusSelector  OutputSignals=SteerOvrCmd,AccelOvrCmd,DecelOvrCmd
  Constant : Constant  Value=false
  Equal Front Rear Bias : Selector  InputPortWidth=1  IndexOptions=Index vector (dialog)  Indices=[1 1]  OutputSizes=1
  Gain : Gain
  Signal Specification : SignalSpecification  Unit=1
  Signal Specification1 : SignalSpecification  Unit=1
  Signal Specification2 : SignalSpecification  Unit=1
  Signal Specification3 : SignalSpecification  Unit=rad
  Signal Specification4 : SignalSpecification  Unit=N*m
  Terminator : Terminator
  Rider : Outport  VectorParamsAs1DForOutWhenUnconnected=off
  wires:
  Signal Specification2/1 -> Bus Creator1/4  "GearCmd"
  Bus Selector1/3 -> Signal Specification1/1  "<DecelOvrCmd>"
  Bus Creator1/1 -> Rider/1
  Bus Selector1/2 -> Signal Specification/1  "<AccelOvrCmd>"
  MotoFdbk/1 -> Terminator/1
  Signal Specification/1 -> Bus Creator1/2  "AccelCmd"
  Equal Front Rear Bias/1 -> Bus Creator1/3  "DecelCmd"
  Constant/1 -> Bus Creator1/5  "IgnSwtch"
  MotoComms/1 -> Bus Selector1/1
  GearCmd/1 -> Signal Specification2/1
  Bus Selector1/1 -> Signal Specification3/1  "<SteerOvrCmd>"
  Signal Specification4/1 -> Bus Creator1/1  "SteerCmd"
  Signal Specification1/1 -> Equal Front Rear Bias/1  "DecelCmd"
  Signal Specification3/1 -> Gain/1
  Gain/1 -> Signal Specification4/1

== system ConfiguredVirtualVehicleModel/Rider Commands/Rider Commands/Predictive Rider ==
  MotoComms : Inport
  MotoFdbk : Inport  Port=2
  Env : Inport  Port=3
  Bus Creator1 : BusCreator  Inputs=5
  Bus Selector : BusSelector  OutputSignals=Body.InertFrm.Cg.Disp.Y,Body.BdyFrm.Cg.Vel.ydot,Body.InertFrm.Cg.Ang.psi,Body.BdyFrm.Cg.AngVel.r
  Bus Selector1 : BusSelector  OutputSignals=LngRef,LtrlRef,EnblSteerCmd,SteerOvrCmd,SteerHld,SteerZero,EnblAccelOvr,AccelOvrCmd,AccelHld,AccelZero,EnblDecelCmd,DecelOvrCmd,DecelHld,DecelZero
  Constant : Constant  Value=false
  Equal Front Rear Bias : Selector  InputPortWidth=1  IndexOptions=Index vector (dialog)  Indices=[1 1]  OutputSizes=1
  Gain : Gain
  Hill Hold : Subsystem
  Linear Predictive Driver : vehdynlibdriver/Predictive Driver  extAccelOvr=on  extDecelOvr=on  extAccelHld=on  extDecelHld=on  extAccelZero=on  extDecelZero=on  extSteerOvr=on  extSteerHld=on  extSteerZero=on  cntrlType=Predictive  cntrlTypeLat=Predictive  shftType=Reverse, Neutral, Drive  coordMode=SAE J670 (Z-down)  refType=Reference pose  velUnits=m/s  angUnits=rad  gearOut=on  steerOut=on  Kp=3  Ki=1  Kff=1  Kg=0  VehVelVec=[0 100]  KffVec=[.1 .1]  KpVec=[10 10]  KiVec=[5 5]  KgVec=[0 0]  vnom=5  Kaw=1  tauerr=.075  tau=DriverTimeConst  L=DriverPreviewDist  Kpt=DriverTractiveForce  aR=DriverRollRes  bR=DriverDrivelineRes  cR=DriverAeroRes  g=EnvGrvty  vecPose=off  dynamMode=off  PositionGainF=2.5  PositionGainR=2.5  YawRateGain=.2  DelayGain=.2  enableDrift=off  BetaRef=10  KpBeta=1  KpDrift=1  KdDrift=1  KpPsi=1  KOmega=.1  tOmega=.1  a=MotoFrmLngth  b=MotoRearArmLngth  m=MotoFrmMass+MotoUpprFrntFrkMass+MotoLowrFrntFrkMass+MotoRearArmMass+RiderMass  Cy_f=DriverFrontCornerStiff  Cy_r=DriverRearCornerStiff  I=MotoFrmInert(3)  Ksteer=1  theta=DriverWheelRange  Idl=1  Re=PlntWhlLdRadius  lambda_mu=1  GearInit=DriverInitialGear  tShift=DriverShiftTime  pdlVec=[0.1 0.4 0.5 0.9]  upShftTbl=[-1 12.9375 26.4375 39.9375 51.18749999999999 62.4375 72.84375 83.25;-1 16.3125 29.8125 43.3125 54.5624 65.8125 76.78125 87.75;-1 19.6875 33.1875 46.68749999999999 57.9375 69.1875 80.71875 92.25;-1 33 52.5 77.25 100.5 138.75 161.875 185]  dwnShftTbl=[-1 12.9375 26.4375 39.9375 51.18749999999999 62.4375 72.84375 83.25;-1 16.3125 29.8125 43.3125 54.5624 65.8125 76.78125 87.75;-1 19.6875 33.1875 46.68749999999999 57.9375 69.1875 80.71875 92.25;-1 33 52.5 77.25 100.5 138.75 161.875 185]  tClutch=.5  tRev=.5  tPark=120  UpGearVec="[0  1  2  3  4  5  6  7]"  DownGearVec="[1  2  3  4  5  6  7  8]"  aMode=2
  Signal Specification4 : SignalSpecification  Unit=N*m
  Terminator : Terminator
  Unit Conversion : UnitConversion
  " Rider" : Outport  VectorParamsAs1DForOutWhenUnconnected=off
  wires:
  Linear Predictive Driver/3 -> Bus Creator1/2  "AccelCmd"
  Bus Selector/2 -> Linear Predictive Driver/18  "<ydot>"
  Bus Selector/1 -> Linear Predictive Driver/17  "<Y>"
  Bus Selector1/10 -> Linear Predictive Driver/10  "<AccelZero>"
  Bus Creator1/1 -> " Rider"/1
  Linear Predictive Driver/1 -> Terminator/1
  Bus Selector/3 -> Linear Predictive Driver/19  "<psi>"
  MotoFdbk/1 -> Hill Hold/7(VehFdbk), Bus Selector/1
  Bus Selector1/2 -> Linear Predictive Driver/2  "<LtrlRef>"
  Bus Selector/4 -> Linear Predictive Driver/20  "<r>"
  MotoComms/1 -> Bus Selector1/1
  Bus Selector1/1 -> Unit Conversion/1  "<LngRef>"
  Signal Specification4/1 -> Bus Creator1/1  "SteerCmd"
  Linear Predictive Driver/4 -> Equal Front Rear Bias/1  "DecelCmd"
  Linear Predictive Driver/5 -> Bus Creator1/4  "GearCmd"
  Constant/1 -> Bus Creator1/5  "IgnSwtch"
  Bus Selector1/3 -> Linear Predictive Driver/3  "<EnblSteerCmd>"
  Bus Selector1/4 -> Linear Predictive Driver/4  "<SteerOvrCmd>"
  Bus Selector1/5 -> Linear Predictive Driver/5  "<SteerHld>"
  Bus Selector1/6 -> Linear Predictive Driver/6  "<SteerZero>"
  Bus Selector1/7 -> Linear Predictive Driver/7  "<EnblAccelOvr>"
  Bus Selector1/8 -> Linear Predictive Driver/8  "<AccelOvrCmd>"
  Bus Selector1/9 -> Linear Predictive Driver/9  "<AccelHld>"
  Bus Selector1/11 -> Hill Hold/2(<EnblDecelCmd>)  "<EnblDecelCmd>"
  Bus Selector1/12 -> Hill Hold/3(<DecelOvrCmd>)  "<DecelOvrCmd>"
  Bus Selector1/13 -> Hill Hold/4(<DecelHld>)  "<DecelHld>"
  Bus Selector1/14 -> Hill Hold/5(<DecelZero>)  "<DecelZero>"
  Env/1 -> Hill Hold/6(Env)
  Hill Hold/5(Grade) -> Linear Predictive Driver/15
  Hill Hold/6(VelFdbk) -> Linear Predictive Driver/16
  Hill Hold/4(DecelZero) -> Linear Predictive Driver/14
  Hill Hold/3(DecelHld) -> Linear Predictive Driver/13
  Hill Hold/2(DecelOvrCmd) -> Linear Predictive Driver/12
  Hill Hold/1(EnblDecelOvr) -> Linear Predictive Driver/11
  Unit Conversion/1 -> Linear Predictive Driver/1, Hill Hold/1(LngRef)
  Equal Front Rear Bias/1 -> Bus Creator1/3  "DecelCmd"
  Gain/1 -> Signal Specification4/1
  Linear Predictive Driver/2 -> Gain/1  "SteerCmd"
